simulink model "Copy_of_fast_powertrain"  (R2020b)
settings: Solver=FixedStepAuto  StartTime=0  StopTime=t(end)  RelTol=1e-3
PreLoadFcn:
  | C_sc = 1;
StartFcn:
  | C_sc = 1;
values from neighbouring files (symbols this model uses):
  fc_power_array = [900 900 900 900 900 900 900 900 900 900 900 900 ... (24566 elements, 71x346)]    [fc_power_climb_dp.mat]    (also in fc_power_cruise_dp.mat = [0 0 0 0 0 0 0 0 0 0 0 0 ... (32589 elements, 71x459)]; fc_power_descend_dp.mat = [285.411057245 285.411057245 285.411057245 285.411057245 285; fc_power_takeoff_dp.mat = [0 0 0 0 0 0 0 0 0 0 0 0 ... (23714 elements, 71x334)])
  Ts = old_data.Ts    [model_fc.m]
undefined symbols (not defined in the file or in its folder): DiscIntNeverNeededParam, Ion, Lithium, w
libraries: neural x50, powerlib x30, fuzblock x7, electricdrivelib x2, lib_converters x2, simulink x1
(part 5 of 5)

== matlab function Copy_of_fast_powertrain/PV MODULE2/PV_function ==
  settings: updateMethod=DISCRETE  sampleTime=Ts
  data: TempCell_C input; ID output; Irradiance input; Ncell input; Voc input; Isc input; Vmp input; Imp input; alpha input; beta input; IPH_STC input; I_0 input; V_PV input; I_PV input; a input; Rp input; Rs input; para_string input; serie_string input
function ID = pv_calculation(TempCell_C, Irradiance, Ncell, Voc, Isc, Vmp, Imp, alpha, beta, IPH_STC, I_0,V_PV, I_PV, a, Rp, Rs, para_string, serie_string)
    %% Constant
    n = a;
    Tc_STC = 25 + 273.15;
    G_STC = 1000;
    TempCell_K = TempCell_C+273.15;
    
    k = 1.3806e-23; % Boltzman constant (J/K)
    k_ = 8.617333262145e-5; % Boltzman constant (eV/K)
    q = 1.602e-19; % Elementary charge on an electron (C)
    % k_ = k/q;
    Eg0 = 1.121;
    Eg_ref = Eg0*q; % Band gap for silicon (eV)
    
    
    

%     
%     if isnan(V_PV)
%         V_PV = 0;
%     end
%     if isnan(I_PV)
%         I_PV = 0;
%     end
    
    
    %% Method 2 + Ncell dans Id + -1 dans Irs + Ish différent
    %     Voc = Voc / Ncell;
    k = 1.3806e-23;
    Vt = k/q*TempCell_K;
    IPH = ((TempCell_K-Tc_STC)*alpha+IPH_STC)*para_string*Irradiance/G_STC;
    Ish = (V_PV + I_PV*Rs)/Rp;
    Irs = IPH_STC/(exp(q*Voc/(Ncell*k*a*TempCell_K))-1);
    Is = Irs * (TempCell_K/Tc_STC)^3*exp((Eg_ref/(k_*a))*(1/TempCell_K - 1/Tc_STC));
    % Maybe change above ? (1/Tc_STC - 1/TempCell_K) ??
    Id = para_string * Is * (exp((V_PV/serie_string+I_PV*Rs/para_string)/(n*Vt*Ncell))-1);
    ID = IPH * para_string - Ish - Id;
    
end


% https://hal.archives-ouvertes.fr/hal-01351308/document
% PV -> autre -> Matlab sim model
% PV -> autre -> PV panel
% PV -> autre -> PV module
% https://environmentalsystemsresearch.springeropen.com/articles/10.1186/s40068-015-0047-9
% https://iopscience.iop.org/article/10.1088/1757-899X/114/1/012137/pdf

== matlab function Copy_of_fast_powertrain/PEMFC matfunc V1/MATLAB Function ==
  settings: updateMethod=DISCRETE  sampleTime=Ts
  data: U_H2 output; U_O2 output; R_ohm output; Ifc input; E_Ner output; E_ohm output; E_con output; E_act_steady output; E_act input; E_act_d output; limit output
function [U_H2,U_O2,R_ohm,E_Ner,E_ohm,E_con,E_act_steady,E_act_d,limit] = fcn(Ifc,E_act)
%     https://link.springer.com/article/10.1007/s40565-016-0196-5
%     Modeling and Simulation of a Proton Exchange Membrane Fuel Cell Alongside a Waste Heat Recovery System Based on the Organic Rankine Cycle in MATLAB/SIMULINK Environment
%     MATHEMATICAL MODELLING FOR PROTON EXCHANGE MEMBRANE FUEL CELL (PEMFC) 
%     https://www.scirp.org/pdf/epe_2020112310053180.pdf#page=17&zoom=100,72,604
%     H-Series Fuel Cell Stacks
% https://ieeexplore.ieee.org/document/6243436
% https://www.scirp.org/journal/paperinformation.aspx?paperid=84317

    %% constants:
    R = 8.3145;
    Pstd = 101325;
    nF = 2*96485;
    C_act = 2;
    A = 19.6*4.0;
    T = 303.15;
    Nfc = 50;
    lambda = 14;
    l = 21e-4 * 10^-2;
%     l = 1.27e-4;
    
    J = Ifc/A;
    JM = 45/A;
    Pa = 1.45;
    Pc = 1;
    Tc = T-273.15;
    coeff = 1.05;
        
%     if Ifc <=0
%         Ifc = 40;
%     end
    
    PH2Osat = 10^(-2.18+2.95e-2*Tc-9.18e-5*Tc^2+1.44e-7*Tc^3);
    
    P_H2 = 0.5*PH2Osat*(exp(-(1.635*J/T^1.334))*(Pa/PH2Osat)-1);
    P_O2 = PH2Osat*(exp(-(4.192*J/T^1.334))*(Pc/PH2Osat)-1);
    

    %% Saturation at start
    if -1.87e-4*log(Ifc) > 0
        k = 0;
    else
        if -1.87e-4*log(Ifc) < -1.2
            k = -1.2;
        else
            k = -1.87e-4*log(Ifc);
        end
    end
    %% Nernst Voltage
    E_Ner = 1.229 + (T-298.15) * (-0.85e-3) + T*R/nF * log(P_H2*P_O2^0.5);
    
    %% Activation loss
    % Pressure not in Pa ?
    CO2 = (P_O2/(5.08e6))*exp(498/T);
%     CH2 = (P_H2/(1.09e6))*exp(-77/T);
%     E_act_steady=-0.9514 + T * (2.86e-3+2.1e-4*log(200)+4.3e-5*log(CH2)+7.4e-5*log(CO2)+k);
    E_act_steady = -0.9514 + 3.12e-3*T + 7.4e-5*T*log(CO2) -1.87e-4*T*log(Ifc);
    
    %% Ohmic loss
%     E_ohm = - Ifc*(l/((lambda*5.139e-3-3.26e-3)*exp(1268*(1/303-1/T))));
    R_ohm = (l/((lambda*5.139e-3-3.26e-3)*exp(1268*(1/303-1/T))));
    E_ohm = -Ifc*l/A*(181.6*(1+0.03*(Ifc/A))+0.062*(T/303)^2*(Ifc/A)^2.5)/((lambda-0.634-3*(Ifc/A))*exp(4.18*((T-303)/T)));
    
    %% Concentration loss
%     if T>= 312.15
%         E_con = (1.1e-4-1.2e-6*(T-273.15))*exp(8*Ifc/40);
%     else
%         E_con = (3.3e-3-8.2e-5*(T-273.15))*exp(8*Ifc/40);
%     end

%     E_con = 3*R*T/(2*nF)*log(1-J/JM)-1.5607*R*T/(2*nF);
    if J/JM < 1
        E_con = 3*R*T/(2*nF)*log(1-J/JM)-1.5607*R*T/(2*nF);
    else
%         E_con = -abs(3*R*T/(2*nF)*log(complex(1-J/(JM-0.001)))-1.5607*R*T/(2*nF));
        E_con = 3*R*T/(2*nF)*log(J/JM)-1.5607*R*T/(2*nF);
    end
    
    %% with coefficient
    E_con = coeff * E_con;
    E_act_steady = coeff * E_act_steady;
    E_ohm = coeff * E_ohm;
    E_Ner = coeff * E_Ner;
    
        
    %% activation dynamic loss:
    below = -E_act_steady-E_con;
    E_act_d = (Ifc/C_act)*(1-E_act/below);
%     E_act_d = 0;

    %% Fuel utilization
    U_H2 = 60000*Ifc*R*T*Nfc/(nF*1.16*1*0.9995*Pstd);
    
    %% Air utilization
    U_O2 = 60000*Ifc*R*T*Nfc/(2*nF*0.0181*1*0.21*Pstd);
    limit = 1;
%     if J/JM >= 1
%             E_con = 0;
%             E_act_steady = 0;
%             E_ohm = 0;
%             E_act_d = 0;
%             E_Ner = -35*Ifc;
%             if E_Ner <= 0
%                 E_Ner = 0;
%             end
%             limit = 0;
%     end
    
    
    %%
end

== matlab function Copy_of_fast_powertrain/SMC ==
  settings: updateMethod=DISCRETE  sampleTime=Ts
  data: Vdc_command input; Vfc input; Ifc_in input; Ifc output; Vfc_conv output; Pload input; I_pv_out input; Vdc_real input; BATT_SOC input; Pbatt_in input
function [Ifc,Vfc_conv] = fcn(Vdc_command,Vfc,Ifc_in, Pload, I_pv_out,Vdc_real, BATT_SOC, Pbatt_in)
    %% FC - control
    % Set / get previous data
    persistent pre_condition;
    if isempty(pre_condition)
        pre_condition=3;
    end
    
    
    % Set boundaries
    % batt
    SOC_min = 40;
    SOC_lb = 50;
    SOC_ub = 80;
    SOC_max = 90;
    
    % fuel cell
    Pfc_min = 100;
    Pfc_rated = 400;
    Pfc_mid = 580;
    Pfc_max = 1100;
    Pfc_command = Pfc_rated;
    
    if Pbatt_in < -200
        alpha = -200-Pbatt_in;
    else
        alpha = 0;
    end
    
    Ppv_out = I_pv_out * Vdc_real;
    Pout = Pload - Ppv_out;

    
    %%  Condition + command
    cur_condition = 3;
    if BATT_SOC < SOC_min
        cur_condition = 1;
    end
    if BATT_SOC >= SOC_min && BATT_SOC < SOC_lb
        cur_condition = pre_condition;
    end
    if BATT_SOC >= SOC_lb && BATT_SOC < SOC_ub
        cur_condition = 2;
    end
    if BATT_SOC >= SOC_ub && BATT_SOC < SOC_max
        cur_condition = pre_condition;
    end
    if BATT_SOC >= SOC_max
        cur_condition = 3;
    end
    
    if cur_condition == 1 && Pout < Pfc_min
        Pfc_command = Pfc_rated; % need to change (get value of the max / typical
        % power to charge the battery)
    end
    if cur_condition == 1 && Pout >= Pfc_min && Pout < Pfc_rated
        Pfc_command = Pfc_rated; % need to change (get value of the max / typical
        % power to charge the battery)
    end
    if cur_condition == 1 && Pout >= Pfc_rated && Pout < Pfc_mid
        Pfc_command = Pfc_max; % need to change (get value of the max / typical
        % power to charge the battery)
    end
    if cur_condition == 1 && Pout >= Pfc_mid && Pout < Pfc_max
        Pfc_command = Pfc_max; % need to change (get value of the max / typical
        % power to charge the battery)
    end
    if cur_condition == 1 && Pout >= Pfc_max
        Pfc_command = Pfc_max;
    end
    
    if cur_condition == 2 && Pout < Pfc_min
        Pfc_command = Pfc_min;
    end
    if cur_condition == 2 && Pout >= Pfc_min && Pout < Pfc_rated
        Pfc_command = Pfc_rated;
    end
    if cur_condition == 2 && Pout >= Pfc_rated && Pout < Pfc_mid
        Pfc_command = Pfc_rated+ (Pfc_mid-Pfc_rated)/4;
    end
    if cur_condition == 2 && Pout >= Pfc_mid && Pout < Pfc_max
        Pfc_command = Pfc_mid;
    end
    if cur_condition == 2 && Pout >= Pfc_max
        Pfc_command = Pfc_mid + (Pfc_max-Pfc_mid)/4;
    end
    
    if cur_condition == 3 && Pout < Pfc_min
        Pfc_command = Pfc_min;
    end
    if cur_condition == 3 && Pout >= Pfc_min && Pout < Pfc_rated
        Pfc_command = Pfc_rated;
    end
    if cur_condition == 3 && Pout >= Pfc_rated && Pout < Pfc_mid
        Pfc_command = Pfc_mid;
    end
    if cur_condition == 3 && Pout >= Pfc_mid && Pout < Pfc_max
        Pfc_command = Pfc_mid + (Pfc_max-Pfc_mid)/2;
    end
    if cur_condition == 3 && Pout >= Pfc_max
        Pfc_command = Pfc_mid + (Pfc_max-Pfc_mid)/4;
    end

    
    Pbatt_diff = 0;
    if (Pout-Pfc_command*0.9)/0.9 > 850
        Pbatt_diff = Pout-800 - 2*alpha;
    end
    if (Pout-Pfc_command*0.9)/0.9 < -150
        Pbatt_diff = Pout-50 - 2*alpha;
    end
    
    Pfc_command = min(1100,max(0,Pfc_command + Pbatt_diff));
    
    
    %% Set output
    % set the pre_condition value:
    pre_condition = cur_condition;
    
    % Converter current command
    Ifc = Pfc_command / Vfc;
    
    % Converter wanted output voltage
    Vfc_conv = Vdc_command;
    if Ifc_in < Ifc
        Vfc_conv = 100;
    end % doesn't work as expected
    
end

== matlab function Copy_of_fast_powertrain/DP ==
  settings: updateMethod=DISCRETE  sampleTime=Ts
  data: Time input; SOC_batt input; Vdc_command input; Ifc_in input; Vfc input; Ifc output; Vfc_conv output; fc_power_array parameter
function [Ifc,Vfc_conv] = fcn(Time, SOC_batt, Vdc_command,Ifc_in, Vfc, fc_power_array)
    soc = 20:1:90;
    persistent Pfc
    if isempty(Pfc)
        Pfc = 0;
    end
    if Time > 1e-3 && ~mod(Time,1)
        [value,index] = min(abs(soc-SOC_batt));
        Pfc = max(0,min(1100,fc_power_array(index,Time)));
    end
    
    % Converter current command
    Ifc = Pfc / Vfc;
    
    % Converter wanted output voltage
    Vfc_conv = Vdc_command;
    if Ifc_in < Ifc
        Vfc_conv = 100;
    end % doesn't work as expected
    
end
